simulink model "scheme5_1"  (R2021a)
settings: Solver=VariableStepAuto  StartTime=0.0  StopTime=30  RelTol=1e-3
values from neighbouring files (symbols this model uses):
  k = 6    [exercise5.m]
  T_1 = 5.1    [exercise5.m]
  T_2 = 0.2    [exercise5.m]
  Td = 0    [exercise5.m]
  Ti = 0.8    [exercise5.m]
undefined symbols (not defined in the file or in its folder): kp
settings Model: Creator=Paweł  LastModifiedBy=Paweł

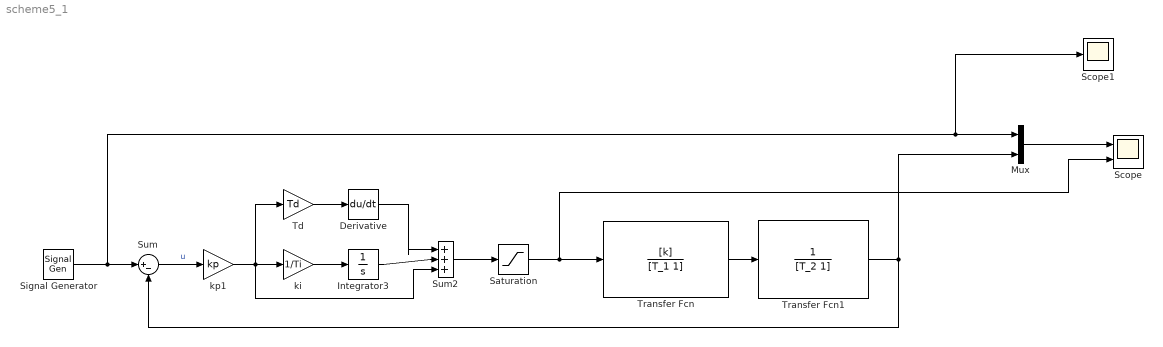
== system scheme5_1 ==
  Derivative : Derivative
  Integrator3 : Integrator
  Mux : Mux  Inputs=2
  Saturation : Saturate  UpperLimit=1  LowerLimit=-1
  Scope : Scope  NumInputPorts=2
  Scope1 : Scope
  Signal Generator : SignalGenerator  WaveForm=square  Frequency=0.1
  Sum : Sum  Inputs=|+-
  Sum2 : Sum  Inputs=|+++  SaturateOnIntegerOverflow=on
  Td : Gain  Gain=Td  SaturateOnIntegerOverflow=on  OutDataTypeStr=Inherit: Same as input  ParamDataTypeStr=Inherit: Same as input
  Transfer Fcn : TransferFcn  Numerator=[k]  Denominator=[T_1 1]
  Transfer Fcn1 : TransferFcn  Denominator=[T_2 1]
  ki : Gain  Gain=1/Ti  SaturateOnIntegerOverflow=on  OutDataTypeStr=Inherit: Same as input  ParamDataTypeStr=Inherit: Same as input
  kp1 : Gain  Gain=kp  SaturateOnIntegerOverflow=on  OutDataTypeStr=Inherit: Same as input  ParamDataTypeStr=Inherit: Same as input
  wires:
  Signal Generator/1 -> Scope1/1, Mux/1, Sum/1
  Derivative/1 -> Sum2/1
  kp1/1 -> Td/1, Sum2/3, ki/1
  ki/1 -> Integrator3/1
  Transfer Fcn/1 -> Transfer Fcn1/1
  Td/1 -> Derivative/1
  Transfer Fcn1/1 -> Sum/2, Mux/2
  Mux/1 -> Scope/1
  Sum/1 -> kp1/1  "u"
  Integrator3/1 -> Sum2/2
  Sum2/1 -> Saturation/1
  Saturation/1 -> Scope/2, Transfer Fcn/1
